simulink model "parma_setup"  (R2015b)
settings: Solver=FixedStepAuto  StartTime=0.0  StopTime=inf  FixedStep=0.1  RelTol=1e-3
undefined symbols (not defined in the file): Position, Position_SL_Info
libraries: robotlib x12, simulink x4, realtime_pacer_lib x1
settings Model: Creator=daniele  LastModifiedBy=daniele

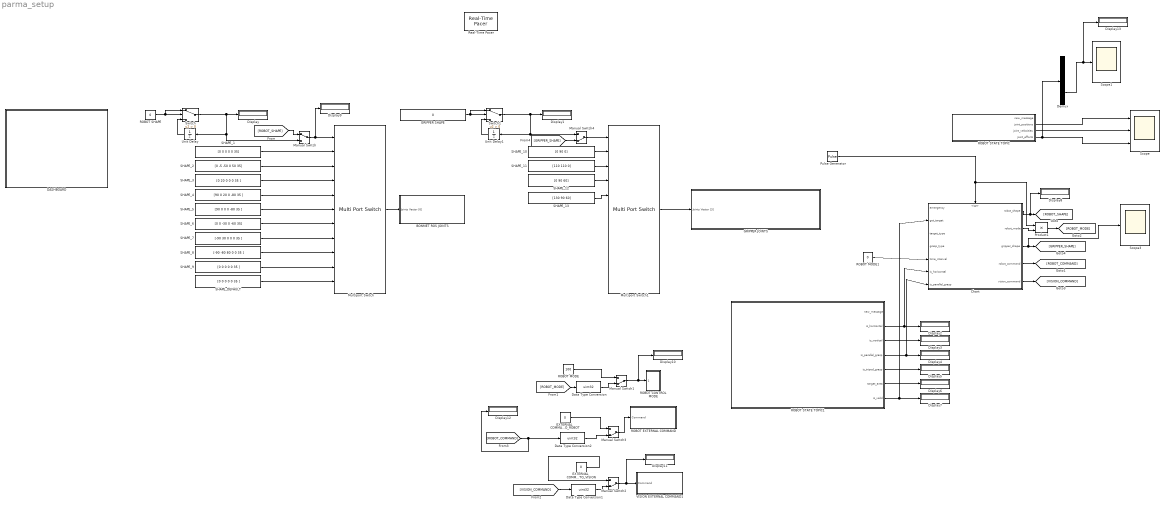
== system parma_setup ==
  BONMET ROS JOINTS : Subsystem
  Chart : Stateflow chart  TreatAsAtomicUnit=on
  DASHBOARD : Subsystem
  Data Type Conversion : DataTypeConversion  OutDataTypeStr=uint32
  Data Type Conversion1 : DataTypeConversion  OutDataTypeStr=uint32
  Data Type Conversion2 : DataTypeConversion  OutDataTypeStr=uint32
  Demux : Demux  Outputs=6
  Display{,1..13} (14 alike) : Display
  "EXTERNAL_COMMAND_TO_ROBOT " : Constant  Value=0  OutDataTypeStr=uint32
  EXTERNAL_COMMAND_TO_VISION : Constant  Value=0  OutDataTypeStr=uint32
  GRIPPER JOINTS : Subsystem
  GRIPPER SHAPE : Constant  Value=0  OutDataTypeStr=double
  Manual Switch : ManualSwitch
  Manual Switch{1..4} (4 alike) : ManualSwitch  CurrentSetting=0
  Multiport Switch : MultiPortSwitch  Inputs=10
  Multiport Switch1 : MultiPortSwitch  Inputs=10
  Product1 : Product
  Pulse Generator : DiscretePulseGenerator  PulseType=Time based  Period=0.7  PulseWidth=50
  ROBOT CONTROL MODE : Subsystem
  ROBOT EXTERNAL COMMAND : Subsystem
  ROBOT MODE : Constant  Value=100  OutDataTypeStr=uint32
  ROBOT MODE1 : Constant  Value=0
  ROBOT SHAPE : Constant  Value=0
  ROBOT STATE TOPIC : Subsystem
  ROBOT STATE TOPIC1 : Subsystem
  Real-Time Pacer : realtime_pacer_lib/Real-Time Pacer  simTimePerRealTime=1
  SHAPE_1 : Constant  Value=[0 0 0 0 0 35]  OutDataTypeStr=double
  SHAPE_10 : Constant  Value=[0 90 0]  OutDataTypeStr=double
  SHAPE_11 : Constant  Value=[110 110 0]  OutDataTypeStr=double
  SHAPE_12 : Constant  Value=[0 90 60]  OutDataTypeStr=double
  SHAPE_13 : Constant  Value=[130 90 60]  OutDataTypeStr=double
  SHAPE_2 : Constant  Value=[0 -5 -50 0 50 35]  OutDataTypeStr=double
  SHAPE_3 : Constant  Value=[0 20 0 0 0 35 ]  OutDataTypeStr=double
  SHAPE_4 : Constant  Value=[90 0 20 0 -80 35 ]  OutDataTypeStr=double
  SHAPE_5 : Constant  Value=[90 0 0 0 -80 35 ]  OutDataTypeStr=double
  SHAPE_6 : Constant  Value=[0 0 -30 0 -60 35]  OutDataTypeStr=double
  SHAPE_7 : Constant  Value=[-90 30 0 0 0 35 ]  OutDataTypeStr=double
  SHAPE_8 : Constant  Value=[-90 -80 80 0 0 35 ]  OutDataTypeStr=double
  SHAPE_9 : Constant  Value=[0 0 0 0 0 35 ]  OutDataTypeStr=double
  SHAPE_DEFAULT : Constant  Value=[0 0 0 0 0 35 ]  OutDataTypeStr=double
  Scope : Scope  NumInputPorts=3
  Scope1 : Scope
  Scope3 : Scope
  Switch : Switch  Criteria=u2 > Threshold
  Switch1 : Switch  Criteria=u2 > Threshold
  Unit Delay : UnitDelay  InitialCondition=1  SampleTime=-1
  Unit Delay1 : UnitDelay  InitialCondition=1  SampleTime=-1
  VISION EXTERNAL COMMAND1 : Subsystem
  wires:
  ROBOT STATE TOPIC/2(joint_positions) -> Scope/1
  SHAPE_1/1 -> Multiport Switch/2
  SHAPE_2/1 -> Multiport Switch/3
  Multiport Switch/1 -> BONMET ROS JOINTS/1(Joints Vector [6])
  Switch/1 -> Display/1, Manual Switch/2, Unit Delay/1
  ROBOT STATE TOPIC/3(joint_velocities) -> Scope/2
  ROBOT STATE TOPIC/4(joint_efforts) -> Demux/1, Scope/3
  SHAPE_3/1 -> Multiport Switch/4
  SHAPE_4/1 -> Multiport Switch/5
  SHAPE_5/1 -> Multiport Switch/6
  SHAPE_6/1 -> Multiport Switch/7
  SHAPE_7/1 -> Multiport Switch/8
  SHAPE_8/1 -> Multiport Switch/9
  SHAPE_9/1 -> Multiport Switch/10
  SHAPE_DEFAULT/1 -> Multiport Switch/11
  ROBOT SHAPE/1 -> Switch/1, Switch/2
  Unit Delay/1 -> Switch/3
  Multiport Switch1/1 -> GRIPPER JOINTS/1(Joints Vector [3])
  SHAPE_10/1 -> Multiport Switch1/2
  SHAPE_11/1 -> Multiport Switch1/3
  Switch1/1 -> Manual Switch4/1, Unit Delay1/1, Display1/1
  GRIPPER SHAPE/1 -> Switch1/1, Switch1/2
  Unit Delay1/1 -> Switch1/3
  EXTERNAL_COMMAND_TO_VISION/1 -> Manual Switch2/1
  SHAPE_12/1 -> Multiport Switch1/4
  SHAPE_13/1 -> Multiport Switch1/5
  ROBOT STATE TOPIC1/2(is_horizontal) -> Chart/6(is_horizontal), Display2/1
  ROBOT STATE TOPIC1/3(is_vertical) -> Display3/1
  ROBOT STATE TOPIC1/4(is_parallel_grasp) -> Chart/7(is_parallel_grasp), Display4/1
  ROBOT STATE TOPIC1/5(is_tripod_grasp) -> Display5/1
  ROBOT STATE TOPIC1/6(target_area) -> Display6/1
  ROBOT STATE TOPIC1/7(is_valid) -> Chart/2(got_target), Display7/1
  Manual Switch/1 -> Display9/1, Multiport Switch/1
  Chart/1(robot_shape) -> Display8/1, [ROBOT_SHAPE]
  [ROBOT_SHAPE] -> Manual Switch/1
  Pulse Generator/1 -> Product1/1, Chart/Trigger
  Chart/4(robot_command) -> [ROBOT_COMMAND]
  ROBOT MODE/1 -> Manual Switch1/1
  [ROBOT_MODE] -> Data Type Conversion/1
  Manual Switch1/1 -> Display10/1, ROBOT CONTROL MODE/1(MODE)
  Data Type Conversion/1 -> Manual Switch1/2
  Product1/1 -> [ROBOT_MODE]
  Chart/2(robot_mode) -> Product1/2
  Chart/5(vision_command) -> [VISION_COMMAND]
  [VISION_COMMAND] -> Data Type Conversion1/1
  Data Type Conversion1/1 -> Manual Switch2/2
  Manual Switch2/1 -> Display11/1, VISION EXTERNAL COMMAND1/1(Command)
  ROBOT MODE1/1 -> Chart/5(time_interval)
  "EXTERNAL_COMMAND_TO_ROBOT "/1 -> Manual Switch3/1
  Manual Switch3/1 -> ROBOT EXTERNAL COMMAND/1(Command)
  [ROBOT_COMMAND] -> Display12/1, Data Type Conversion2/1
  Data Type Conversion2/1 -> Manual Switch3/2
  Chart/3(gripper_shape) -> Scope3/1, [GRIPPER_SHAPE]
  [GRIPPER_SHAPE] -> Manual Switch4/2
  Manual Switch4/1 -> Multiport Switch1/1
  Demux/5 -> Display13/1, Scope1/1

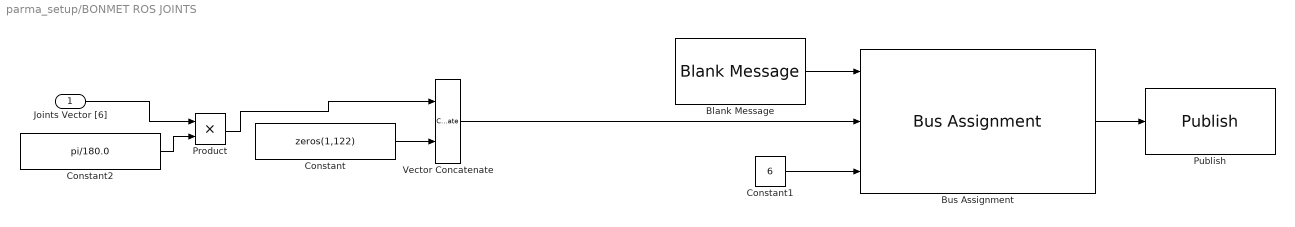
== system parma_setup/BONMET ROS JOINTS ==
  Joints Vector [6] : Inport
  Blank Message : robotlib/Blank Message  SourceLibraryInfo=This block requires Robotics System Toolbox  messageType=sensor_msgs/JointState  SampleTime=inf
  Bus Assignment : BusAssignment  AssignedSignals=Position,Position_SL_Info.CurrentLength
  Constant : Constant  Value=zeros(1,122)
  Constant1 : Constant  Value=6  OutDataTypeStr=uint32
  Constant2 : Constant  Value=pi/180.0
  Product : Product
  Publish : robotlib/Publish  SourceLibraryInfo=This block requires Robotics System Toolbox  topicSource=Select from ROS network  topic=/bonmetc60/joint_command  messageType=sensor_msgs/JointState  messageQueueLength=1
  Vector Concatenate : Concatenate
  wires:
  Bus Assignment/1 -> Publish/1
  Constant1/1 -> Bus Assignment/3
  Vector Concatenate/1 -> Bus Assignment/2
  Blank Message/1 -> Bus Assignment/1
  Constant/1 -> Vector Concatenate/2
  Constant2/1 -> Product/2
  Joints Vector [6]/1 -> Product/1
  Product/1 -> Vector Concatenate/1

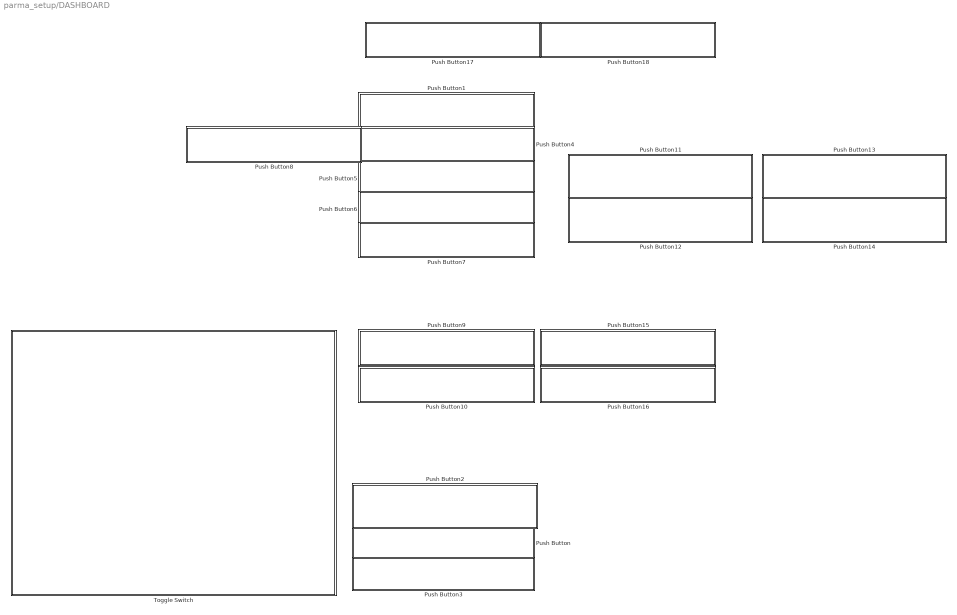
== system parma_setup/DASHBOARD ==
  Push Button : Subsystem  DialogController=hmiCreateDDGDialog  IsWebBlock=on  mask(MWDashboardBlock){webBlockId=a14e1f79-182e-44d4-a7bb-5d0475f1f540, webBlockType=pushbutton, ShowInLibBrwoser=on, ShowInitialText=on, HMISrcModelName=BONMET_TEST}
      mask prompts: webBlockId "WebBlock Id"; webBlockType "WebBlock Type"; HMISrcModelName "Source Model"
      mask Help: helpview([docroot '/mapfiles/simulink.map'], 'hmi_push_button')
      mask Display:
      | model = bdroot(gcb);
      | if strcmp(get_param(model,'BlockDiagramType'), 'library')
      |     image([(matlabroot) '/toolbox/simulink/hmi/icons/PushButton.png']);
      | end
  Push Button1 : Subsystem  DialogController=hmiCreateDDGDialog  IsWebBlock=on  mask(MWDashboardBlock){webBlockId=48464d7c-7824-4a1e-a082-c1efe53c48b9, webBlockType=pushbutton, ShowInLibBrwoser=on, ShowInitialText=on, HMISrcModelName=BONMET_TEST}
      mask prompts: webBlockId "WebBlock Id"; webBlockType "WebBlock Type"; HMISrcModelName "Source Model"
      mask Help: helpview([docroot '/mapfiles/simulink.map'], 'hmi_push_button')
      mask Display:
      | model = bdroot(gcb);
      | if strcmp(get_param(model,'BlockDiagramType'), 'library')
      |     image([(matlabroot) '/toolbox/simulink/hmi/icons/PushButton.png']);
      | end
  Push Button10 : Subsystem  DialogController=hmiCreateDDGDialog  IsWebBlock=on  mask(MWDashboardBlock){webBlockId=3147c314-1eab-453b-9dc2-aca05f0efa20, webBlockType=pushbutton, ShowInLibBrwoser=on, ShowInitialText=on, HMISrcModelName=BONMET_TEST}
      mask prompts: webBlockId "WebBlock Id"; webBlockType "WebBlock Type"; HMISrcModelName "Source Model"
      mask Help: helpview([docroot '/mapfiles/simulink.map'], 'hmi_push_button')
      mask Display:
      | model = bdroot(gcb);
      | if strcmp(get_param(model,'BlockDiagramType'), 'library')
      |     image([(matlabroot) '/toolbox/simulink/hmi/icons/PushButton.png']);
      | end
  Push Button11 : Subsystem  DialogController=hmiCreateDDGDialog  IsWebBlock=on  mask(MWDashboardBlock){webBlockId=f5a10ce5-d5f9-4e6b-a437-c8a656b22730, webBlockType=pushbutton, ShowInLibBrwoser=on, ShowInitialText=on, HMISrcModelName=BONMET_TEST}
      mask prompts: webBlockId "WebBlock Id"; webBlockType "WebBlock Type"; HMISrcModelName "Source Model"
      mask Help: helpview([docroot '/mapfiles/simulink.map'], 'hmi_push_button')
      mask Display:
      | model = bdroot(gcb);
      | if strcmp(get_param(model,'BlockDiagramType'), 'library')
      |     image([(matlabroot) '/toolbox/simulink/hmi/icons/PushButton.png']);
      | end
  Push Button12 : Subsystem  DialogController=hmiCreateDDGDialog  IsWebBlock=on  mask(MWDashboardBlock){webBlockId=cf6e00d0-e9fd-4913-890a-2af90d875abb, webBlockType=pushbutton, ShowInLibBrwoser=on, ShowInitialText=on, HMISrcModelName=BONMET_TEST}
      mask prompts: webBlockId "WebBlock Id"; webBlockType "WebBlock Type"; HMISrcModelName "Source Model"
      mask Help: helpview([docroot '/mapfiles/simulink.map'], 'hmi_push_button')
      mask Display:
      | model = bdroot(gcb);
      | if strcmp(get_param(model,'BlockDiagramType'), 'library')
      |     image([(matlabroot) '/toolbox/simulink/hmi/icons/PushButton.png']);
      | end
  Push Button13 : Subsystem  DialogController=hmiCreateDDGDialog  IsWebBlock=on  mask(MWDashboardBlock){webBlockId=b731ab2c-3ee8-4e4b-a288-873d5cd90223, webBlockType=pushbutton, ShowInLibBrwoser=on, ShowInitialText=on, HMISrcModelName=BONMET_TEST}
      mask prompts: webBlockId "WebBlock Id"; webBlockType "WebBlock Type"; HMISrcModelName "Source Model"
      mask Help: helpview([docroot '/mapfiles/simulink.map'], 'hmi_push_button')
      mask Display:
      | model = bdroot(gcb);
      | if strcmp(get_param(model,'BlockDiagramType'), 'library')
      |     image([(matlabroot) '/toolbox/simulink/hmi/icons/PushButton.png']);
      | end
  Push Button14 : Subsystem  DialogController=hmiCreateDDGDialog  IsWebBlock=on  mask(MWDashboardBlock){webBlockId=a37e7b4a-4bb1-4f91-bfbf-bec0431e08be, webBlockType=pushbutton, ShowInLibBrwoser=on, ShowInitialText=on, HMISrcModelName=BONMET_TEST}
      mask prompts: webBlockId "WebBlock Id"; webBlockType "WebBlock Type"; HMISrcModelName "Source Model"
      mask Help: helpview([docroot '/mapfiles/simulink.map'], 'hmi_push_button')
      mask Display:
      | model = bdroot(gcb);
      | if strcmp(get_param(model,'BlockDiagramType'), 'library')
      |     image([(matlabroot) '/toolbox/simulink/hmi/icons/PushButton.png']);
      | end
  Push Button15 : Subsystem  DialogController=hmiCreateDDGDialog  IsWebBlock=on  mask(MWDashboardBlock){webBlockId=6e041370-8963-4a95-af56-4df54b493523, webBlockType=pushbutton, ShowInLibBrwoser=on, ShowInitialText=on, HMISrcModelName=BONMET_TEST}
      mask prompts: webBlockId "WebBlock Id"; webBlockType "WebBlock Type"; HMISrcModelName "Source Model"
      mask Help: helpview([docroot '/mapfiles/simulink.map'], 'hmi_push_button')
      mask Display:
      | model = bdroot(gcb);
      | if strcmp(get_param(model,'BlockDiagramType'), 'library')
      |     image([(matlabroot) '/toolbox/simulink/hmi/icons/PushButton.png']);
      | end
  Push Button16 : Subsystem  DialogController=hmiCreateDDGDialog  IsWebBlock=on  mask(MWDashboardBlock){webBlockId=bb8cf605-0616-45d0-bab8-a325ac824327, webBlockType=pushbutton, ShowInLibBrwoser=on, ShowInitialText=on, HMISrcModelName=BONMET_TEST}
      mask prompts: webBlockId "WebBlock Id"; webBlockType "WebBlock Type"; HMISrcModelName "Source Model"
      mask Help: helpview([docroot '/mapfiles/simulink.map'], 'hmi_push_button')
      mask Display:
      | model = bdroot(gcb);
      | if strcmp(get_param(model,'BlockDiagramType'), 'library')
      |     image([(matlabroot) '/toolbox/simulink/hmi/icons/PushButton.png']);
      | end
  Push Button17 : Subsystem  DialogController=hmiCreateDDGDialog  IsWebBlock=on  mask(MWDashboardBlock){webBlockId=adba6b7a-b0cd-426f-8bf6-e7efb589b193, webBlockType=pushbutton, ShowInLibBrwoser=on, ShowInitialText=on, HMISrcModelName=BONMET_TEST}
      mask prompts: webBlockId "WebBlock Id"; webBlockType "WebBlock Type"; HMISrcModelName "Source Model"
      mask Help: helpview([docroot '/mapfiles/simulink.map'], 'hmi_push_button')
      mask Display:
      | model = bdroot(gcb);
      | if strcmp(get_param(model,'BlockDiagramType'), 'library')
      |     image([(matlabroot) '/toolbox/simulink/hmi/icons/PushButton.png']);
      | end
  Push Button18 : Subsystem  DialogController=hmiCreateDDGDialog  IsWebBlock=on  mask(MWDashboardBlock){webBlockId=dd331435-0126-45c5-8987-ed7f02f039cf, webBlockType=pushbutton, ShowInLibBrwoser=on, ShowInitialText=on, HMISrcModelName=BONMET_TEST}
      mask prompts: webBlockId "WebBlock Id"; webBlockType "WebBlock Type"; HMISrcModelName "Source Model"
      mask Help: helpview([docroot '/mapfiles/simulink.map'], 'hmi_push_button')
      mask Display:
      | model = bdroot(gcb);
      | if strcmp(get_param(model,'BlockDiagramType'), 'library')
      |     image([(matlabroot) '/toolbox/simulink/hmi/icons/PushButton.png']);
      | end
  Push Button2 : Subsystem  DialogController=hmiCreateDDGDialog  IsWebBlock=on  mask(MWDashboardBlock){webBlockId=ffedc718-3234-4d76-b6e1-84798166140b, webBlockType=pushbutton, ShowInLibBrwoser=on, ShowInitialText=on, HMISrcModelName=BONMET_TEST}
      mask prompts: webBlockId "WebBlock Id"; webBlockType "WebBlock Type"; HMISrcModelName "Source Model"
      mask Help: helpview([docroot '/mapfiles/simulink.map'], 'hmi_push_button')
      mask Display:
      | model = bdroot(gcb);
      | if strcmp(get_param(model,'BlockDiagramType'), 'library')
      |     image([(matlabroot) '/toolbox/simulink/hmi/icons/PushButton.png']);
      | end
  Push Button3 : Subsystem  DialogController=hmiCreateDDGDialog  IsWebBlock=on  mask(MWDashboardBlock){webBlockId=0634655a-ca9c-45e0-acf0-95d5b4921e02, webBlockType=pushbutton, ShowInLibBrwoser=on, ShowInitialText=on, HMISrcModelName=BONMET_TEST}
      mask prompts: webBlockId "WebBlock Id"; webBlockType "WebBlock Type"; HMISrcModelName "Source Model"
      mask Help: helpview([docroot '/mapfiles/simulink.map'], 'hmi_push_button')
      mask Display:
      | model = bdroot(gcb);
      | if strcmp(get_param(model,'BlockDiagramType'), 'library')
      |     image([(matlabroot) '/toolbox/simulink/hmi/icons/PushButton.png']);
      | end
  Push Button4 : Subsystem  DialogController=hmiCreateDDGDialog  IsWebBlock=on  mask(MWDashboardBlock){webBlockId=3477ac38-8f96-421b-ad45-2305eb4e464c, webBlockType=pushbutton, ShowInLibBrwoser=on, ShowInitialText=on, HMISrcModelName=BONMET_TEST}
      mask prompts: webBlockId "WebBlock Id"; webBlockType "WebBlock Type"; HMISrcModelName "Source Model"
      mask Help: helpview([docroot '/mapfiles/simulink.map'], 'hmi_push_button')
      mask Display:
      | model = bdroot(gcb);
      | if strcmp(get_param(model,'BlockDiagramType'), 'library')
      |     image([(matlabroot) '/toolbox/simulink/hmi/icons/PushButton.png']);
      | end
  Push Button5 : Subsystem  DialogController=hmiCreateDDGDialog  IsWebBlock=on  mask(MWDashboardBlock){webBlockId=407b7faa-dac7-4f3e-b193-e73c9785f71c, webBlockType=pushbutton, ShowInLibBrwoser=on, ShowInitialText=on, HMISrcModelName=BONMET_TEST}
      mask prompts: webBlockId "WebBlock Id"; webBlockType "WebBlock Type"; HMISrcModelName "Source Model"
      mask Help: helpview([docroot '/mapfiles/simulink.map'], 'hmi_push_button')
      mask Display:
      | model = bdroot(gcb);
      | if strcmp(get_param(model,'BlockDiagramType'), 'library')
      |     image([(matlabroot) '/toolbox/simulink/hmi/icons/PushButton.png']);
      | end
  Push Button6 : Subsystem  DialogController=hmiCreateDDGDialog  IsWebBlock=on  mask(MWDashboardBlock){webBlockId=f5817f0e-87ec-44fc-bd82-9f81bf8a9dc3, webBlockType=pushbutton, ShowInLibBrwoser=on, ShowInitialText=on, HMISrcModelName=BONMET_TEST}
      mask prompts: webBlockId "WebBlock Id"; webBlockType "WebBlock Type"; HMISrcModelName "Source Model"
      mask Help: helpview([docroot '/mapfiles/simulink.map'], 'hmi_push_button')
      mask Display:
      | model = bdroot(gcb);
      | if strcmp(get_param(model,'BlockDiagramType'), 'library')
      |     image([(matlabroot) '/toolbox/simulink/hmi/icons/PushButton.png']);
      | end
  Push Button7 : Subsystem  DialogController=hmiCreateDDGDialog  IsWebBlock=on  mask(MWDashboardBlock){webBlockId=4738a42b-1085-4b1e-80a7-4467a1327011, webBlockType=pushbutton, ShowInLibBrwoser=on, ShowInitialText=on, HMISrcModelName=BONMET_TEST}
      mask prompts: webBlockId "WebBlock Id"; webBlockType "WebBlock Type"; HMISrcModelName "Source Model"
      mask Help: helpview([docroot '/mapfiles/simulink.map'], 'hmi_push_button')
      mask Display:
      | model = bdroot(gcb);
      | if strcmp(get_param(model,'BlockDiagramType'), 'library')
      |     image([(matlabroot) '/toolbox/simulink/hmi/icons/PushButton.png']);
      | end
  Push Button8 : Subsystem  DialogController=hmiCreateDDGDialog  IsWebBlock=on  mask(MWDashboardBlock){webBlockId=40b70e35-9e89-4285-a460-393df57ddec6, webBlockType=pushbutton, ShowInLibBrwoser=on, ShowInitialText=on, HMISrcModelName=BONMET_TEST}
      mask prompts: webBlockId "WebBlock Id"; webBlockType "WebBlock Type"; HMISrcModelName "Source Model"
      mask Help: helpview([docroot '/mapfiles/simulink.map'], 'hmi_push_button')
      mask Display:
      | model = bdroot(gcb);
      | if strcmp(get_param(model,'BlockDiagramType'), 'library')
      |     image([(matlabroot) '/toolbox/simulink/hmi/icons/PushButton.png']);
      | end
  Push Button9 : Subsystem  DialogController=hmiCreateDDGDialog  IsWebBlock=on  mask(MWDashboardBlock){webBlockId=58f14154-f8a5-499f-b94c-44757bd10921, webBlockType=pushbutton, ShowInLibBrwoser=on, ShowInitialText=on, HMISrcModelName=BONMET_TEST}
      mask prompts: webBlockId "WebBlock Id"; webBlockType "WebBlock Type"; HMISrcModelName "Source Model"
      mask Help: helpview([docroot '/mapfiles/simulink.map'], 'hmi_push_button')
      mask Display:
      | model = bdroot(gcb);
      | if strcmp(get_param(model,'BlockDiagramType'), 'library')
      |     image([(matlabroot) '/toolbox/simulink/hmi/icons/PushButton.png']);
      | end
  Toggle Switch : Subsystem  DialogController=hmiCreateDDGDialog  IsWebBlock=on  mask(MWDashboardBlock){webBlockId=bd00f813-5598-4a74-8fec-42e79a924e80, webBlockType=toggleswitch, ShowInLibBrowser=on, ShowInitialText=on, HMISrcModelName=BONMET_TEST}
      mask prompts: webBlockId "WebBlock Id"; webBlockType "WebBlock Type"; HMISrcModelName "Source Model"
      mask Help: helpview([docroot '/mapfiles/simulink.map'], 'hmi_toggle_switch')
      mask Display:
      | if strcmp(get_param(bdroot(gcb),'BlockDiagramType'), 'library')
      |     image([(matlabroot) '/toolbox/simulink/hmi/icons/ToggleSwitch.png']);
      | end

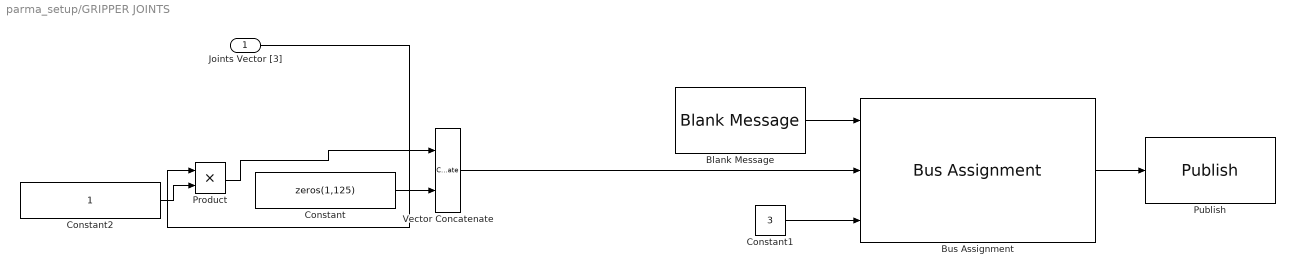
== system parma_setup/GRIPPER JOINTS ==
  Joints Vector [3] : Inport
  Blank Message : robotlib/Blank Message  SourceLibraryInfo=This block requires Robotics System Toolbox  messageType=sensor_msgs/JointState  SampleTime=inf
  Bus Assignment : BusAssignment  AssignedSignals=Position,Position_SL_Info.CurrentLength
  Constant : Constant  Value=zeros(1,125)
  Constant1 : Constant  Value=3  OutDataTypeStr=uint32
  Constant2 : Constant
  Product : Product
  Publish : robotlib/Publish  SourceLibraryInfo=This block requires Robotics System Toolbox  topicSource=Select from ROS network  topic=/trifinger2/joint_command  messageType=sensor_msgs/JointState  messageQueueLength=1
  Vector Concatenate : Concatenate
  wires:
  Constant/1 -> Vector Concatenate/2
  Joints Vector [3]/1 -> Product/1
  Product/1 -> Vector Concatenate/1
  Vector Concatenate/1 -> Bus Assignment/2
  Blank Message/1 -> Bus Assignment/1
  Constant1/1 -> Bus Assignment/3
  Constant2/1 -> Product/2
  Bus Assignment/1 -> Publish/1

== system parma_setup/ROBOT CONTROL MODE ==
  MODE : Inport
  " ROBOT CONTROL MODE TOPIC " : Subsystem
  Change Detecotr : Subsystem
  wires:
  MODE/1 -> Change Detecotr/1(data), " ROBOT CONTROL MODE TOPIC "/1(MODE)
  Change Detecotr/1(changed?) -> " ROBOT CONTROL MODE TOPIC "/Trigger

== system parma_setup/ROBOT EXTERNAL COMMAND ==
  Command : Inport
  Change Detecotr : Subsystem
  ROBOT EXTERNAL COMMAND TOPIC : Subsystem
  wires:
  Command/1 -> ROBOT EXTERNAL COMMAND TOPIC/1(Command), Change Detecotr/1(data)
  Change Detecotr/1(changed?) -> ROBOT EXTERNAL COMMAND TOPIC/Trigger

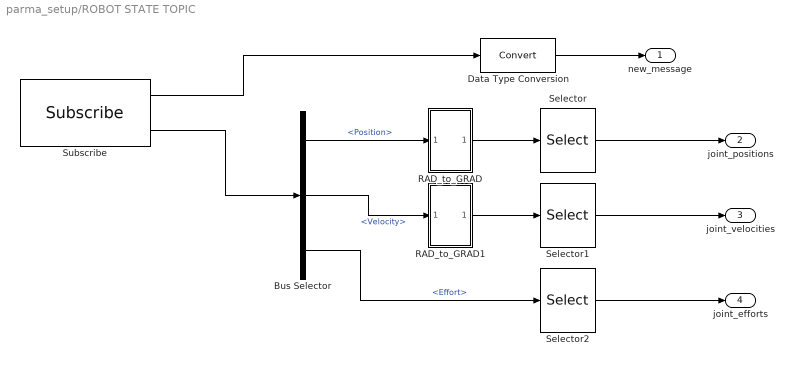
== system parma_setup/ROBOT STATE TOPIC ==
  Bus Selector : BusSelector  OutputSignals=Position,Velocity,Effort
  Data Type Conversion : DataTypeConversion
  RAD_to_GRAD : Subsystem
  RAD_to_GRAD1 : Subsystem
  Selector : Selector  InputPortWidth=128  IndexOptions=Starting index (dialog)  Indices=[1]  OutputSizes=6
  Selector1 : Selector  InputPortWidth=128  IndexOptions=Starting index (dialog)  Indices=[1]  OutputSizes=6
  Selector2 : Selector  InputPortWidth=128  IndexOptions=Starting index (dialog)  Indices=[1]  OutputSizes=6
  Subscribe : robotlib/Subscribe  SourceLibraryInfo=This block requires Robotics System Toolbox  topicSource=Select from ROS network  topic=/bonmetc60/joint_state  messageType=sensor_msgs/JointState  sampleTime=-1  messageQueueLength=1
  new_message : Outport
  joint_positions : Outport  Port=2
  joint_velocities : Outport  Port=3
  joint_efforts : Outport  Port=4
  wires:
  Subscribe/2 -> Bus Selector/1
  Selector/1 -> joint_positions/1
  Subscribe/1 -> Data Type Conversion/1
  Data Type Conversion/1 -> new_message/1
  Bus Selector/1 -> RAD_to_GRAD/1(rad)  "<Position>"
  RAD_to_GRAD/1("grad ") -> Selector/1
  Bus Selector/2 -> RAD_to_GRAD1/1(rad)  "<Velocity>"
  RAD_to_GRAD1/1("grad ") -> Selector1/1
  Selector1/1 -> joint_velocities/1
  Bus Selector/3 -> Selector2/1  "<Effort>"
  Selector2/1 -> joint_efforts/1

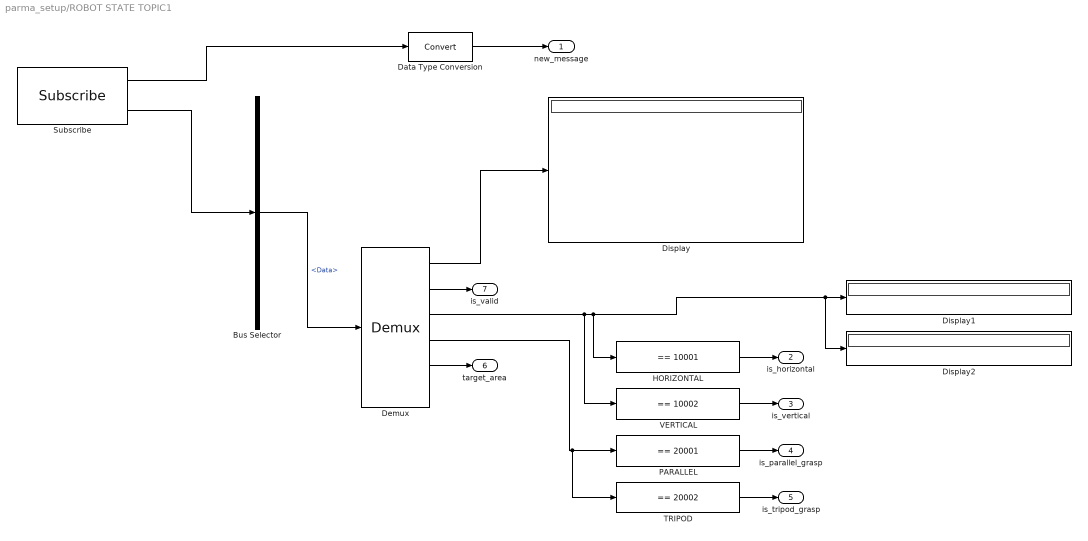
== system parma_setup/ROBOT STATE TOPIC1 ==
  Bus Selector : BusSelector  OutputSignals=Data
  Data Type Conversion : DataTypeConversion
  Demux : Demux  Outputs=[16 1 1 1 1 108]
  Display : Display
  Display1 : Display
      settings: Format=decimal (Stored Integer)
  Display2 : Display
      settings: Format=decimal (Stored Integer)
  HORIZONTAL : simulink/Logic and Bit Operations/Compare To Constant  relop===  const=10001  OutDataTypeStr=uint8
  PARALLEL : simulink/Logic and Bit Operations/Compare To Constant  relop===  const=20001  OutDataTypeStr=uint8
  Subscribe : robotlib/Subscribe  SourceLibraryInfo=This block requires Robotics System Toolbox  topicSource=Select from ROS network  topic=/vision_system/object_target_info  messageType=std_msgs/Float32MultiArray  sampleTime=-1  messageQueueLength=1
  TRIPOD : simulink/Logic and Bit Operations/Compare To Constant  relop===  const=20002  OutDataTypeStr=uint8
  VERTICAL : simulink/Logic and Bit Operations/Compare To Constant  relop===  const=10002  OutDataTypeStr=uint8
  new_message : Outport
  is_horizontal : Outport  Port=2
  is_vertical : Outport  Port=3
  is_parallel_grasp : Outport  Port=4
  is_tripod_grasp : Outport  Port=5
  target_area : Outport  Port=6
  is_valid : Outport  Port=7
  wires:
  Data Type Conversion/1 -> new_message/1
  Subscribe/1 -> Data Type Conversion/1
  Subscribe/2 -> Bus Selector/1
  Bus Selector/1 -> Demux/1  "<Data>"
  Demux/1 -> Display/1
  HORIZONTAL/1 -> is_horizontal/1
  VERTICAL/1 -> is_vertical/1
  PARALLEL/1 -> is_parallel_grasp/1
  TRIPOD/1 -> is_tripod_grasp/1
  Demux/2 -> is_valid/1
  Demux/3 -> VERTICAL/1, HORIZONTAL/1, Display2/1, Display1/1
  Demux/5 -> target_area/1
  Demux/4 -> TRIPOD/1, PARALLEL/1

== system parma_setup/VISION EXTERNAL COMMAND1 ==
  Command : Inport
  Change Detecotr : Subsystem
  ROBOT EXTERNAL COMMAND TOPIC : Subsystem
  wires:
  Command/1 -> ROBOT EXTERNAL COMMAND TOPIC/1(Command), Change Detecotr/1(data)
  Change Detecotr/1(changed?) -> ROBOT EXTERNAL COMMAND TOPIC/Trigger

== system parma_setup/DASHBOARD/Push Button ==

== system parma_setup/DASHBOARD/Push Button1 ==

== system parma_setup/DASHBOARD/Push Button10 ==

== system parma_setup/DASHBOARD/Push Button11 ==

== system parma_setup/DASHBOARD/Push Button12 ==

== system parma_setup/DASHBOARD/Push Button13 ==

== system parma_setup/DASHBOARD/Push Button14 ==

== system parma_setup/DASHBOARD/Push Button15 ==

== system parma_setup/DASHBOARD/Push Button16 ==

== system parma_setup/DASHBOARD/Push Button17 ==

== system parma_setup/DASHBOARD/Push Button18 ==

== system parma_setup/DASHBOARD/Push Button2 ==

== system parma_setup/DASHBOARD/Push Button3 ==

== system parma_setup/DASHBOARD/Push Button4 ==

== system parma_setup/DASHBOARD/Push Button5 ==

== system parma_setup/DASHBOARD/Push Button6 ==

== system parma_setup/DASHBOARD/Push Button7 ==

== system parma_setup/DASHBOARD/Push Button8 ==

== system parma_setup/DASHBOARD/Push Button9 ==

== system parma_setup/DASHBOARD/Toggle Switch ==

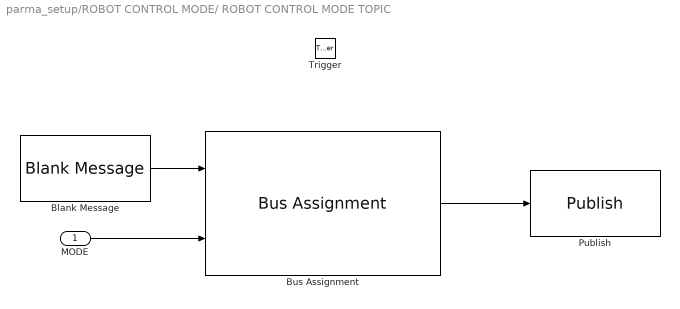
== system parma_setup/ROBOT CONTROL MODE/ ROBOT CONTROL MODE TOPIC  ==
  MODE : Inport
  Trigger : TriggerPort  PortDimensions=1
  Blank Message : robotlib/Blank Message  SourceLibraryInfo=This block requires Robotics System Toolbox  messageType=std_msgs/UInt32  SampleTime=inf
  Bus Assignment : BusAssignment  AssignedSignals=Data
  Publish : robotlib/Publish  SourceLibraryInfo=This block requires Robotics System Toolbox  topicSource=Select from ROS network  topic=/bonmetc60/mode_command  messageType=std_msgs/UInt32  messageQueueLength=1
  wires:
  Bus Assignment/1 -> Publish/1
  Blank Message/1 -> Bus Assignment/1
  MODE/1 -> Bus Assignment/2

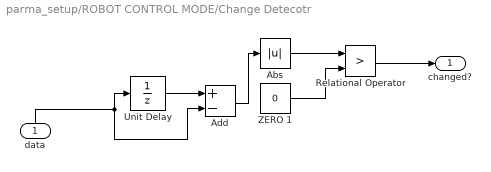
== system parma_setup/ROBOT CONTROL MODE/Change Detecotr ==
  data : Inport
  Abs : Abs
  Add : Sum  Inputs=+-
  Relational Operator : RelationalOperator  Operator=>  OutDataTypeStr=boolean
  Unit Delay : UnitDelay  SampleTime=-1
  ZERO 1 : Constant  Value=0  OutDataTypeStr=uint32
  changed? : Outport
  wires:
  Unit Delay/1 -> Add/1
  Abs/1 -> Relational Operator/1
  Add/1 -> Abs/1
  data/1 -> Add/2, Unit Delay/1
  ZERO 1/1 -> Relational Operator/2
  Relational Operator/1 -> changed?/1

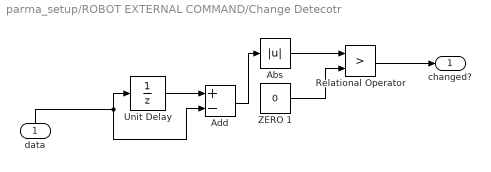
== system parma_setup/ROBOT EXTERNAL COMMAND/Change Detecotr ==
  data : Inport
  Abs : Abs
  Add : Sum  Inputs=+-
  Relational Operator : RelationalOperator  Operator=>  OutDataTypeStr=boolean
  Unit Delay : UnitDelay  SampleTime=-1
  ZERO 1 : Constant  Value=0  OutDataTypeStr=uint32
  changed? : Outport
  wires:
  Unit Delay/1 -> Add/1
  Abs/1 -> Relational Operator/1
  Add/1 -> Abs/1
  data/1 -> Add/2, Unit Delay/1
  ZERO 1/1 -> Relational Operator/2
  Relational Operator/1 -> changed?/1

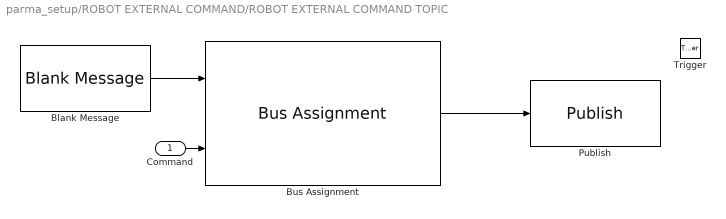
== system parma_setup/ROBOT EXTERNAL COMMAND/ROBOT EXTERNAL COMMAND TOPIC ==
  Command : Inport
  Trigger : TriggerPort  PortDimensions=1
  Blank Message : robotlib/Blank Message  SourceLibraryInfo=This block requires Robotics System Toolbox  messageType=std_msgs/UInt32  SampleTime=inf
  Bus Assignment : BusAssignment  AssignedSignals=Data
  Publish : robotlib/Publish  SourceLibraryInfo=This block requires Robotics System Toolbox  topicSource=Select from ROS network  topic=/bonmetc60/external_command  messageType=std_msgs/UInt32  messageQueueLength=1
  wires:
  Blank Message/1 -> Bus Assignment/1
  Bus Assignment/1 -> Publish/1
  Command/1 -> Bus Assignment/2

== system parma_setup/ROBOT STATE TOPIC/RAD_to_GRAD ==
  rad : Inport
  Constant3 : Constant  Value=180/pi  OutDataTypeStr=uint32
  Product : Product
  "grad " : Outport
  wires:
  Constant3/1 -> Product/2
  rad/1 -> Product/1
  Product/1 -> "grad "/1

== system parma_setup/ROBOT STATE TOPIC/RAD_to_GRAD1 ==
  rad : Inport
  Constant3 : Constant  Value=180/pi  OutDataTypeStr=uint32
  Product : Product
  "grad " : Outport
  wires:
  Product/1 -> "grad "/1
  rad/1 -> Product/1
  Constant3/1 -> Product/2

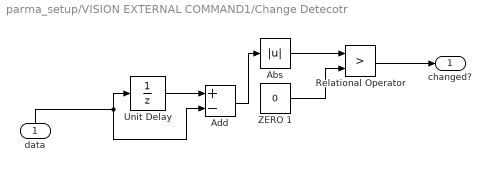
== system parma_setup/VISION EXTERNAL COMMAND1/Change Detecotr ==
  data : Inport
  Abs : Abs
  Add : Sum  Inputs=+-
  Relational Operator : RelationalOperator  Operator=>  OutDataTypeStr=boolean
  Unit Delay : UnitDelay  SampleTime=-1
  ZERO 1 : Constant  Value=0  OutDataTypeStr=uint32
  changed? : Outport
  wires:
  Unit Delay/1 -> Add/1
  Abs/1 -> Relational Operator/1
  Add/1 -> Abs/1
  data/1 -> Add/2, Unit Delay/1
  ZERO 1/1 -> Relational Operator/2
  Relational Operator/1 -> changed?/1

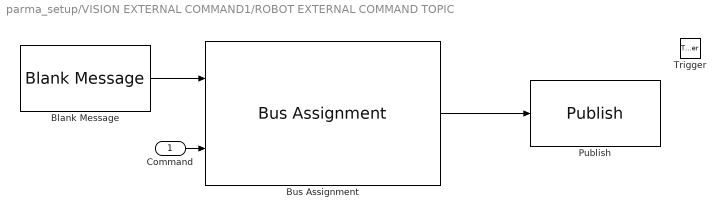
== system parma_setup/VISION EXTERNAL COMMAND1/ROBOT EXTERNAL COMMAND TOPIC ==
  Command : Inport
  Trigger : TriggerPort  PortDimensions=1
  Blank Message : robotlib/Blank Message  SourceLibraryInfo=This block requires Robotics System Toolbox  messageType=std_msgs/UInt32  SampleTime=inf
  Bus Assignment : BusAssignment  AssignedSignals=Data
  Publish : robotlib/Publish  SourceLibraryInfo=This block requires Robotics System Toolbox  topicSource=Select from ROS network  topic=/vision_system/external_command  messageType=std_msgs/UInt32  messageQueueLength=1
  wires:
  Blank Message/1 -> Bus Assignment/1
  Bus Assignment/1 -> Publish/1
  Command/1 -> Bus Assignment/2

== stateflow chart parma_setup/Chart ==
  state ROBOT_SYNC1
    entry:
    wait_counter=5
    robot_command=ROBOT_COMMAND_SYNC
  state NO_TARGET
    entry:
    robot_shape=1
    gripper_shape=1
    vision_command=0
    robot_mode=100
  state TARGET_HORIZONTAL
    entry:
    robot_shape=6
  state GOT_TARGET
    entry:
    wait_counter=time_interval
  state TARGET_VERTICAL
    entry: robot_shape=2
  state WAIT
    entry: wait_counter=wait_counter-1
  state ROBOT_SYNC
    entry:
    wait_counter=time_interval
    robot_command=ROBOT_COMMAND_SYNC
  state ROBOT_DESYNC3
    entry:
    robot_command=0
  state OPEN_GRIPPER_PARALLEL
    entry:
    gripper_shape=1
  state FAR_POSITION1
    entry:
    robot_mode=105
    vision_command=10104
    wait_counter=time_interval
  state OPEN_GRIPPER_TRIPOD
    entry:
    gripper_shape=3
  state VOID
    entry:
  state WAIT3
    entry: wait_counter=wait_counter-1
  state ROBOT_SYNC2
    entry:
    wait_counter=time_interval
    robot_command=ROBOT_COMMAND_SYNC
  state ROBOT_DESYNC1
    entry:
    robot_command=0
  state NEAR_POSITION
    entry:
    robot_mode=105
    vision_command=10103
    wait_counter=time_interval
  state WAIT4
    entry: wait_counter=wait_counter-1
  state ROBOT_SYNC3
    entry:
    wait_counter=time_interval
    robot_command=ROBOT_COMMAND_SYNC
  state CLOSE_GRIPPER_PARALLEL
    entry:
    gripper_shape=2
  state ROBOT_DESYNC2
    entry:
    robot_command=0
  state CLOSE_GRIPPER
    entry:
    robot_mode=105
    vision_command=10103
    wait_counter=time_interval
  state CLOSE_GRIPPER_TRIPOD
    entry:
    gripper_shape=4
  state WAIT5
    entry: wait_counter=wait_counter-1
  state ROBOT_SYNC4
    entry:
    wait_counter=time_interval
    robot_command=ROBOT_COMMAND_SYNC
  state ROBOT_DESYNC
    entry:
    robot_command=0
  state FAR_POSITION
    entry:
    robot_mode=105
    vision_command=10104
    wait_counter=time_interval
  state WAIT6
    entry: wait_counter=wait_counter-1
  state ROBOT_SYNC5
    entry:
    wait_counter=time_interval
    robot_command=ROBOT_COMMAND_SYNC
  state ROBOT_DESYNC7
    entry:
    robot_command=0
  state OBJECT_GRASPED
  state TARGET_HORIZONTAL1
    entry:
    robot_shape=6
    robot_mode=100
  state TARGET_VERTICAL1
    entry: robot_shape=2
    robot_mode=100
  state OBJECT_GRASPED1
    entry: vision_command=10003
  state WAIT7
    entry: wait_counter=wait_counter-1
  state ROBOT_SYNC6
    entry:
    wait_counter=time_interval
    robot_command=ROBOT_COMMAND_SYNC
  state ROBOT_DESYNC4
    entry:
    robot_command=0
  state BOX_POSITION
    entry:
    robot_mode=100
    robot_shape=4
    wait_counter=time_interval
  state WAIT8
    entry: wait_counter=wait_counter-1
  state ROBOT_SYNC7
    entry:
    wait_counter=time_interval
    robot_command=ROBOT_COMMAND_SYNC
  state OPEN_GRIPPER_PARALLEL1
    entry:
    gripper_shape=1
  state ROBOT_DESYNC5
    entry:
    robot_command=0
  state OPEN_GRIPPER1
    entry:
    robot_mode=100
    robot_shape=1
    wait_counter=time_interval
  state CLOSE_GRIPPER_TRIPOD1
    entry:
    gripper_shape=3
  state WAIT9
    entry: wait_counter=wait_counter-1
  state ROBOT_SYNC8
    entry:
    wait_counter=time_interval
    robot_command=ROBOT_COMMAND_SYNC
  state ROBOT_DESYNC6
    entry:
    robot_command=0
  ROBOT_DESYNC6 -> NO_TARGET
  (default) -> NO_TARGET
  NO_TARGET -> ROBOT_SYNC1 [order 2]
  ROBOT_SYNC1 -> NO_TARGET
  NO_TARGET -> GOT_TARGET [order 1] : [got_target==1]
  GOT_TARGET -> TARGET_HORIZONTAL [order 1] : [is_horizontal==1]
  TARGET_HORIZONTAL -> WAIT
  GOT_TARGET -> TARGET_VERTICAL [order 2] : [is_horizontal==0]
  TARGET_VERTICAL -> WAIT
  WAIT -> WAIT [order 1] : [wait_counter>0]
  WAIT -> ROBOT_SYNC [order 2]
  ROBOT_SYNC -> ROBOT_DESYNC3
  FAR_POSITION1 -> OPEN_GRIPPER_PARALLEL [order 1] : [is_parallel_grasp==1]
  ROBOT_DESYNC3 -> FAR_POSITION1
  OPEN_GRIPPER_PARALLEL -> VOID
  FAR_POSITION1 -> OPEN_GRIPPER_TRIPOD [order 2] : [is_parallel_grasp==0]
  OPEN_GRIPPER_TRIPOD -> VOID
  VOID -> WAIT3
  WAIT3 -> WAIT3 [order 1] : [wait_counter>0]
  WAIT3 -> ROBOT_SYNC2 [order 2]
  ROBOT_SYNC2 -> ROBOT_DESYNC1
  ROBOT_DESYNC1 -> NEAR_POSITION
  NEAR_POSITION -> WAIT4
  WAIT4 -> WAIT4 [order 1] : [wait_counter>0]
  WAIT4 -> ROBOT_SYNC3 [order 2]
  ROBOT_SYNC3 -> ROBOT_DESYNC2
  CLOSE_GRIPPER -> CLOSE_GRIPPER_PARALLEL [order 1] : [is_parallel_grasp==1]
  ROBOT_DESYNC2 -> CLOSE_GRIPPER
  CLOSE_GRIPPER_PARALLEL -> WAIT5
  CLOSE_GRIPPER -> CLOSE_GRIPPER_TRIPOD [order 2] : [is_parallel_grasp==0]
  CLOSE_GRIPPER_TRIPOD -> WAIT5
  WAIT5 -> WAIT5 [order 1] : [wait_counter>0]
  WAIT5 -> ROBOT_SYNC4 [order 2]
  ROBOT_SYNC4 -> ROBOT_DESYNC
  ROBOT_DESYNC -> FAR_POSITION
  FAR_POSITION -> WAIT6
  WAIT6 -> WAIT6 [order 1] : [wait_counter>0]
  WAIT6 -> ROBOT_SYNC5 [order 2]
  ROBOT_SYNC5 -> ROBOT_DESYNC7
  ROBOT_DESYNC7 -> OBJECT_GRASPED
  OBJECT_GRASPED -> TARGET_HORIZONTAL1 [order 1] : [is_horizontal==1]
  OBJECT_GRASPED -> TARGET_VERTICAL1 [order 2] : [is_horizontal==0]
  TARGET_HORIZONTAL1 -> OBJECT_GRASPED1
  TARGET_VERTICAL1 -> OBJECT_GRASPED1
  OBJECT_GRASPED1 -> WAIT7
  WAIT7 -> WAIT7 [order 1] : [wait_counter>0]
  WAIT7 -> ROBOT_SYNC6 [order 2]
  ROBOT_SYNC6 -> ROBOT_DESYNC4
  ROBOT_DESYNC4 -> BOX_POSITION
  BOX_POSITION -> WAIT8
  WAIT8 -> WAIT8 [order 1] : [wait_counter>0]
  WAIT8 -> ROBOT_SYNC7 [order 2]
  ROBOT_SYNC7 -> ROBOT_DESYNC5
  OPEN_GRIPPER1 -> OPEN_GRIPPER_PARALLEL1 [order 1] : [is_parallel_grasp==1]
  ROBOT_DESYNC5 -> OPEN_GRIPPER1
  OPEN_GRIPPER_PARALLEL1 -> WAIT9
  OPEN_GRIPPER1 -> CLOSE_GRIPPER_TRIPOD1 [order 2] : [is_parallel_grasp==0]
  CLOSE_GRIPPER_TRIPOD1 -> WAIT9
  WAIT9 -> WAIT9 [order 1] : [wait_counter>0]
  WAIT9 -> ROBOT_SYNC8 [order 2]
  ROBOT_SYNC8 -> ROBOT_DESYNC6
  data: robot_shape output size=1 =1; robot_mode output =100; gripper_shape output size=1 =1; robot_command output size=1 =1; vision_command output size=1; emergency input; got_target input; target_type input; grasp_type input; time_interval input; wait_counter local; ROBOT_COMMAND_SYNC constant double =1010; is_horizontal input; is_parallel_grasp input
  events: trigger input RISING_EDGE_EVENT
